simulink model "Cold_Storage_Final"  (R2018a)
settings: Solver=VariableStepAuto  StartTime=0.0  StopTime=5000  RelTol=1e-3
libraries: simulink x2
settings Model: Creator=BALUCH  LastModifiedBy=BALUCH
settings DataIOCC: ReturnWorkspaceOutputs=on
settings SFSimCC: SimUseLocalCustomCode=on
settings RTWCC: RTWUseLocalCustomCode=on

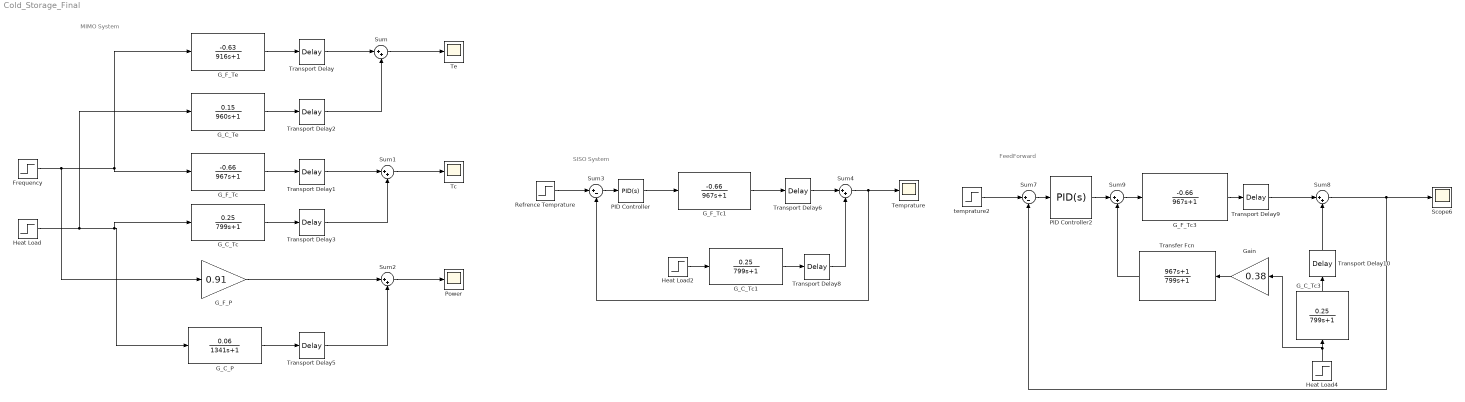
== system Cold_Storage_Final ==
  note: MIMO System
  note: SISO System
  note: FeedForward
  Frequency : Step  Time=60  SampleTime=0
  G_C_P : TransferFcn  Numerator=[0.06]  Denominator=[1341 1]
  G_C_Tc : TransferFcn  Numerator=[0.25]  Denominator=[799 1]
  G_C_Tc1 : TransferFcn  Numerator=[0.25]  Denominator=[799 1]
  G_C_Tc3 : TransferFcn  Numerator=[0.25]  Denominator=[799 1]
  G_C_Te : TransferFcn  Numerator=[0.15]  Denominator=[960 1]
  G_F_P : Gain  Gain=0.91
  G_F_Tc : TransferFcn  Numerator=[-0.66]  Denominator=[967 1]
  G_F_Tc1 : TransferFcn  Numerator=[-0.66]  Denominator=[967 1]
  G_F_Tc3 : TransferFcn  Numerator=[-0.66]  Denominator=[967 1]
  G_F_Te : TransferFcn  Numerator=[-0.63]  Denominator=[916 1]
  Gain : Gain  Gain=0.38
  Heat Load : Step  Time=10  SampleTime=0
  Heat Load2 : Step  Time=0  SampleTime=0
  Heat Load4 : Step  Time=0  After=1400  SampleTime=0
  PID Controller : simulink/Continuous/PID Controller  Controller=PID  Form=Parallel  TimeDomain=Continuous-time  SampleTime=-1  IntegratorMethod=Forward Euler  FilterMethod=Forward Euler  ControllerParametersSource=internal  P=-50.23  I=0.011  D=14  UseFilter=on  N=10000  TunerSelectOption=Transfer Function Based (PID Tuner App)  InitialConditionSource=internal  InitialConditionForIntegrator=0  InitialConditionForFilter=0  DifferentiatorICPrevScaledInput=0  ExternalReset=none  TrackingMode=off  Kt=1  LimitOutput=off  UpperSaturationLimit=inf  LowerSaturationLimit=-inf  LinearizeAsGain=on  AntiWindupMode=none  Kb=1  POutMin=[]  POutMax=[]  IOutMin=[]  IOutMax=[]  DOutMin=[]  DOutMax=[]  NOutMin=[]  NOutMax=[]  SumOutMin=[]  SumOutMax=[]  SaturationOutMin=[]  SaturationOutMax=[]  PParamMin=[]  PParamMax=[]  IParamMin=[]  IParamMax=[]  DParamMin=[]  DParamMax=[]  NParamMin=[]  NParamMax=[]  KbParamMin=[]  KbParamMax=[]  KtParamMin=[]  KtParamMax=[]  KbOutMin=[]  KbOutMax=[]  KtOutMin=[]  KtOutMax=[]  IntegratorOutMin=[]  IntegratorOutMax=[]  FilterOutMin=[]  FilterOutMax=[]  SumI1OutMin=[]  SumI1OutMax=[]  SumI2OutMin=[]  SumI2OutMax=[]  SumI3OutMin=[]  SumI3OutMax=[]  SumDOutMin=[]  SumDOutMax=[]  DifferentiatorOutMin=[]  DifferentiatorOutMax=[]  FilterDiffOutCoefMin=[]  FilterDiffOutCoefMax=[]  ReciprocalOutMin=[]  ReciprocalOutMax=[]  SumDenOutMin=[]  SumDenOutMax=[]  SumNumOutMin=[]  SumNumOutMax=[]  DivideOutMin=[]  DivideOutMax=[]  IntegratorContinuousStateAttributes=''  IntegratorStateMustResolveToSignalObject=off  IntegratorRTWStateStorageClass=Auto  FilterContinuousStateAttributes=''  FilterStateMustResolveToSignalObject=off  FilterRTWStateStorageClass=Auto
  PID Controller2 : simulink/Continuous/PID Controller  Controller=PID  Form=Parallel  TimeDomain=Continuous-time  SampleTime=-1  IntegratorMethod=Forward Euler  FilterMethod=Forward Euler  ControllerParametersSource=internal  P=-50.23  I=0.011  D=14  UseFilter=on  N=1000  TunerSelectOption=Transfer Function Based (PID Tuner App)  InitialConditionSource=internal  InitialConditionForIntegrator=0  InitialConditionForFilter=0  DifferentiatorICPrevScaledInput=0  ExternalReset=none  TrackingMode=off  Kt=1  LimitOutput=off  UpperSaturationLimit=inf  LowerSaturationLimit=-inf  LinearizeAsGain=on  AntiWindupMode=none  Kb=1  POutMin=[]  POutMax=[]  IOutMin=[]  IOutMax=[]  DOutMin=[]  DOutMax=[]  NOutMin=[]  NOutMax=[]  SumOutMin=[]  SumOutMax=[]  SaturationOutMin=[]  SaturationOutMax=[]  PParamMin=[]  PParamMax=[]  IParamMin=[]  IParamMax=[]  DParamMin=[]  DParamMax=[]  NParamMin=[]  NParamMax=[]  KbParamMin=[]  KbParamMax=[]  KtParamMin=[]  KtParamMax=[]  KbOutMin=[]  KbOutMax=[]  KtOutMin=[]  KtOutMax=[]  IntegratorOutMin=[]  IntegratorOutMax=[]  FilterOutMin=[]  FilterOutMax=[]  SumI1OutMin=[]  SumI1OutMax=[]  SumI2OutMin=[]  SumI2OutMax=[]  SumI3OutMin=[]  SumI3OutMax=[]  SumDOutMin=[]  SumDOutMax=[]  DifferentiatorOutMin=[]  DifferentiatorOutMax=[]  FilterDiffOutCoefMin=[]  FilterDiffOutCoefMax=[]  ReciprocalOutMin=[]  ReciprocalOutMax=[]  SumDenOutMin=[]  SumDenOutMax=[]  SumNumOutMin=[]  SumNumOutMax=[]  DivideOutMin=[]  DivideOutMax=[]  IntegratorContinuousStateAttributes=''  IntegratorStateMustResolveToSignalObject=off  IntegratorRTWStateStorageClass=Auto  FilterContinuousStateAttributes=''  FilterStateMustResolveToSignalObject=off  FilterRTWStateStorageClass=Auto
  Power : Scope
  Refrence Temprature : Step  Time=0  After=5  SampleTime=0
  Scope6 : Scope
  Sum{,1..2,4,8..9} (6 alike) : Sum  Inputs=|++
  Sum3 : Sum  Inputs=|+-
  Sum7 : Sum  Inputs=|+-
  Tc : Scope
  Te : Scope
  Temprature : Scope
  Transfer Fcn : TransferFcn  Numerator=[967 1]  Denominator=[799 1]
  Transport Delay{,3,8,10} (4 alike) : TransportDelay  DelayTime=15
  Transport Delay1 : TransportDelay  DelayTime=35
  Transport Delay2 : TransportDelay  DelayTime=42
  Transport Delay5 : TransportDelay  DelayTime=182
  Transport Delay6 : TransportDelay  DelayTime=35
  Transport Delay9 : TransportDelay  DelayTime=35
  temprature2 : Step  Time=0  After=5  SampleTime=0
  wires:
  Sum2/1 -> Power/1
  Sum/1 -> Te/1
  Sum1/1 -> Tc/1
  G_C_Tc/1 -> Transport Delay3/1
  G_C_P/1 -> Transport Delay5/1
  G_F_P/1 -> Sum2/1
  Transport Delay5/1 -> Sum2/2
  G_F_Tc/1 -> Transport Delay1/1
  Transport Delay3/1 -> Sum1/2
  G_C_Te/1 -> Transport Delay2/1
  Heat Load/1 -> G_C_P/1, G_C_Tc/1, G_C_Te/1
  Transport Delay1/1 -> Sum1/1
  Frequency/1 -> G_F_Tc/1, G_F_Te/1, G_F_P/1
  Transport Delay2/1 -> Sum/2
  Transport Delay/1 -> Sum/1
  G_F_Te/1 -> Transport Delay/1
  Sum4/1 -> Temprature/1, Sum3/2
  Heat Load2/1 -> G_C_Tc1/1
  Sum3/1 -> PID Controller/1
  PID Controller/1 -> G_F_Tc1/1
  Refrence Temprature/1 -> Sum3/1
  G_C_Tc1/1 -> Transport Delay8/1
  Transport Delay8/1 -> Sum4/2
  G_F_Tc1/1 -> Transport Delay6/1
  Transport Delay6/1 -> Sum4/1
  Sum7/1 -> PID Controller2/1
  Transport Delay10/1 -> Sum8/2
  temprature2/1 -> Sum7/1
  Transport Delay9/1 -> Sum8/1
  G_F_Tc3/1 -> Transport Delay9/1
  Sum8/1 -> Scope6/1, Sum7/2
  G_C_Tc3/1 -> Transport Delay10/1
  PID Controller2/1 -> Sum9/1
  Sum9/1 -> G_F_Tc3/1
  Transfer Fcn/1 -> Sum9/2
  Gain/1 -> Transfer Fcn/1
  Heat Load4/1 -> Gain/1, G_C_Tc3/1
